simulink model "Model_3RC_P0"  (R2022b)
settings: Solver=FixedStepAuto  StartTime=0.0  StopTime=10000  FixedStep=1  RelTol=1e-3
undefined symbols (not defined in the file): epsilon, OCV, OCV_offset, R0, R1, R2, R3, SOC_levels, tau1, tau2, tau3
settings Model: Creator=frederikvanmaele  LastModifiedBy=AdministratorDevice
settings DebuggingCC: UnconnectedInputMsg=warning  UnconnectedOutputMsg=warning  UnconnectedLineMsg=warning
settings ModelReferenceCC: EnableRefExpFcnMdlSchedulingChecks=on
settings RTWCC: DLArmComputeVersion=19.05

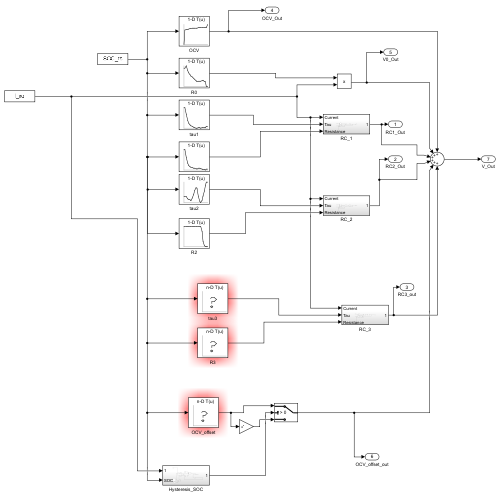
[thumbnail: Simulink's stored preview of the top-level diagram]
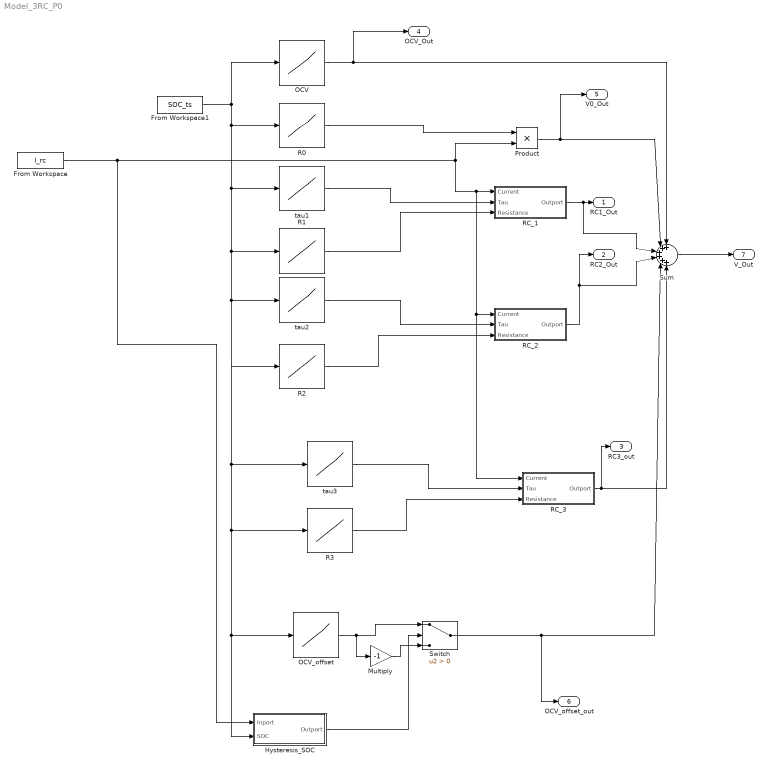
== system Model_3RC_P0 ==
  From Workspace : FromWorkspace  VariableName=I_rc
  From Workspace1 : FromWorkspace  VariableName=SOC_ts
  Hysteresis_SOC : Subsystem
  Multiply : Gain  Gain=-1
  OCV : Lookup_n-D  NumberOfTableDimensions=1  BreakpointsForDimension1=SOC_levels  BeginIndexSearchUsingPreviousIndexResult=on  Table=OCV  UseLastTableValue=on  InternalRulePriority=Speed  OutDataTypeStr=Inherit: Inherit via back propagation  RndMeth=Simplest
  OCV_offset : Lookup_n-D  NumberOfTableDimensions=1  BreakpointsForDimension1=SOC_levels  Table=OCV_offset  InternalRulePriority=Speed  RndMeth=Simplest
  Product : Product
  R0 : Lookup_n-D  NumberOfTableDimensions=1  BreakpointsForDimension1=SOC_levels  BeginIndexSearchUsingPreviousIndexResult=on  Table=R0  ExtrapMethod=Clip  UseLastTableValue=on  InternalRulePriority=Speed  RndMeth=Simplest
  R1 : Lookup_n-D  NumberOfTableDimensions=1  BreakpointsForDimension1=SOC_levels  BeginIndexSearchUsingPreviousIndexResult=on  Table=R1  ExtrapMethod=Clip  UseLastTableValue=on  InternalRulePriority=Speed  RndMeth=Simplest
  R2 : Lookup_n-D  NumberOfTableDimensions=1  BreakpointsForDimension1=SOC_levels  BeginIndexSearchUsingPreviousIndexResult=on  Table=R2  ExtrapMethod=Clip  UseLastTableValue=on  InternalRulePriority=Speed  RndMeth=Simplest
  R3 : Lookup_n-D  NumberOfTableDimensions=1  BreakpointsForDimension1=SOC_levels  BeginIndexSearchUsingPreviousIndexResult=on  Table=R3  ExtrapMethod=Clip  UseLastTableValue=on  InternalRulePriority=Speed  RndMeth=Simplest
  RC_1 : Subsystem
  RC_2 : Subsystem
  RC_3 : Subsystem
  Sum : Sum  Inputs=++++++
  Switch : Switch  Criteria=u2 > Threshold  SaturateOnIntegerOverflow=off  InputSameDT=off
  tau1 : Lookup_n-D  NumberOfTableDimensions=1  BreakpointsForDimension1=SOC_levels  BeginIndexSearchUsingPreviousIndexResult=on  Table=tau1  ExtrapMethod=Clip  UseLastTableValue=on  InternalRulePriority=Speed  RndMeth=Simplest
  tau2 : Lookup_n-D  NumberOfTableDimensions=1  BreakpointsForDimension1=SOC_levels  BeginIndexSearchUsingPreviousIndexResult=on  Table=tau2  ExtrapMethod=Clip  UseLastTableValue=on  InternalRulePriority=Speed  RndMeth=Simplest
  tau3 : Lookup_n-D  NumberOfTableDimensions=1  BreakpointsForDimension1=SOC_levels  BeginIndexSearchUsingPreviousIndexResult=on  Table=tau3  ExtrapMethod=Clip  UseLastTableValue=on  InternalRulePriority=Speed  RndMeth=Simplest
  RC1_Out : Outport
  RC2_Out : Outport  Port=2
  RC3_out : Outport  Port=3
  OCV_Out : Outport  Port=4
  V0_Out : Outport  Port=5
  OCV_offset_out : Outport  Port=6
  V_Out : Outport  Port=7
  wires:
  R1/1 -> RC_1/3(Resistance)
  tau1/1 -> RC_1/2(Tau)
  RC_1/1(Outport) -> Sum/3, RC1_Out/1
  R2/1 -> RC_2/3(Resistance)
  RC_2/1(Outport) -> RC2_Out/1, Sum/4
  OCV/1 -> OCV_Out/1, Sum/1
  Sum/1 -> V_Out/1
  From Workspace1/1 -> tau3/1, R3/1, Hysteresis_SOC/2(SOC), OCV_offset/1, R1/1, R2/1, tau2/1, tau1/1, R0/1, OCV/1
  R0/1 -> Product/1
  Product/1 -> V0_Out/1, Sum/2
  tau2/1 -> RC_2/2(Tau)
  Multiply/1 -> Switch/3
  Hysteresis_SOC/1(Outport) -> Switch/2
  OCV_offset/1 -> Multiply/1, Switch/1
  Switch/1 -> Sum/5, OCV_offset_out/1
  R3/1 -> RC_3/3(Resistance)
  tau3/1 -> RC_3/2(Tau)
  From Workspace/1 -> Hysteresis_SOC/1(Inport), RC_1/1(Current), RC_3/1(Current), RC_2/1(Current), Product/2
  RC_3/1(Outport) -> RC3_out/1, Sum/6

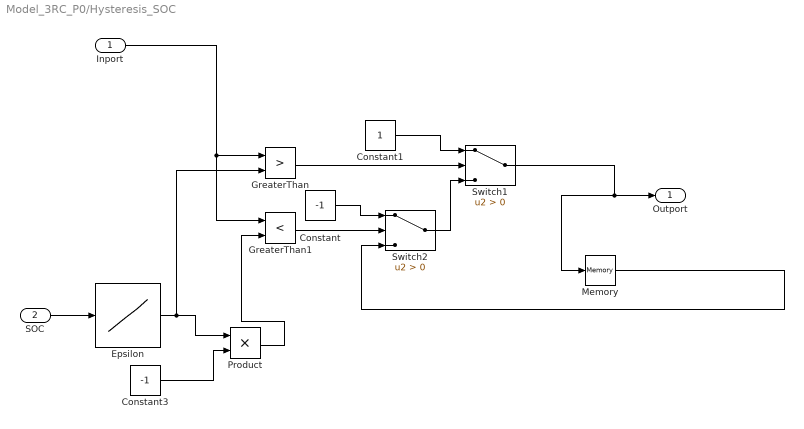
== system Model_3RC_P0/Hysteresis_SOC ==
  Inport : Inport
  SOC : Inport  Port=2
  Constant : Constant  Value=-1
  Constant1 : Constant
  Constant3 : Constant  Value=-1
  Epsilon : Lookup_n-D  NumberOfTableDimensions=1  BreakpointsForDimension1=SOC_levels  Table=epsilon  InternalRulePriority=Speed  RndMeth=Simplest
  GreaterThan : RelationalOperator  Operator=>  OutDataTypeStr=boolean  RndMeth=Simplest  InputSameDT=off
  GreaterThan1 : RelationalOperator  Operator=<  OutDataTypeStr=boolean  RndMeth=Simplest  InputSameDT=off
  Memory : Memory
  Product : Product
  Switch1 : Switch  Criteria=u2 > Threshold  SaturateOnIntegerOverflow=off  InputSameDT=off
  Switch2 : Switch  Criteria=u2 > Threshold  SaturateOnIntegerOverflow=off  InputSameDT=off
  Outport : Outport
  wires:
  GreaterThan1/1 -> Switch2/2
  Constant/1 -> Switch2/1
  Switch1/1 -> Outport/1, Memory/1
  Inport/1 -> GreaterThan1/1, GreaterThan/1
  Constant1/1 -> Switch1/1
  Switch2/1 -> Switch1/3
  GreaterThan/1 -> Switch1/2
  Memory/1 -> Switch2/3
  SOC/1 -> Epsilon/1
  Epsilon/1 -> GreaterThan/2, Product/1
  Constant3/1 -> Product/2
  Product/1 -> GreaterThan1/2

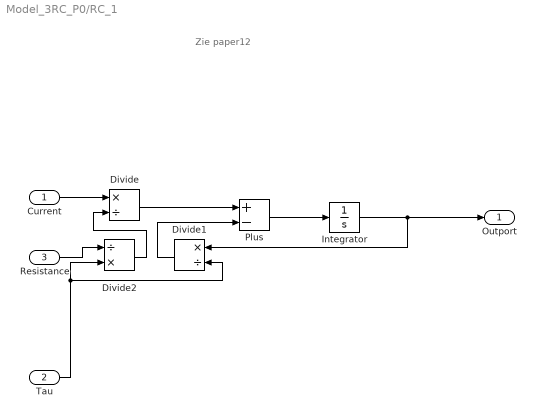
== system Model_3RC_P0/RC_1 ==
  note: Zie paper12
  Current : Inport
  Tau : Inport  Port=2
  Resistance : Inport  Port=3
  Divide : Product  Inputs=*/
  Divide1 : Product  Inputs=*/
  Divide2 : Product  Inputs=/*
  Integrator : Integrator
  Plus : Sum  Inputs=+-
  Outport : Outport
  wires:
  Tau/1 -> Divide2/2, Divide1/2
  Divide/1 -> Plus/1
  Plus/1 -> Integrator/1
  Current/1 -> Divide/1
  Divide1/1 -> Plus/2
  Resistance/1 -> Divide2/1
  Divide2/1 -> Divide/2
  Integrator/1 -> Divide1/1, Outport/1

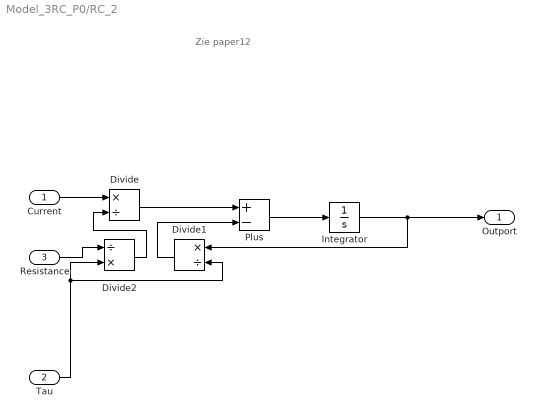
== system Model_3RC_P0/RC_2 ==
  note: Zie paper12
  Current : Inport
  Tau : Inport  Port=2
  Resistance : Inport  Port=3
  Divide : Product  Inputs=*/
  Divide1 : Product  Inputs=*/
  Divide2 : Product  Inputs=/*
  Integrator : Integrator
  Plus : Sum  Inputs=+-
  Outport : Outport
  wires:
  Tau/1 -> Divide2/2, Divide1/2
  Divide/1 -> Plus/1
  Plus/1 -> Integrator/1
  Current/1 -> Divide/1
  Divide1/1 -> Plus/2
  Resistance/1 -> Divide2/1
  Divide2/1 -> Divide/2
  Integrator/1 -> Divide1/1, Outport/1

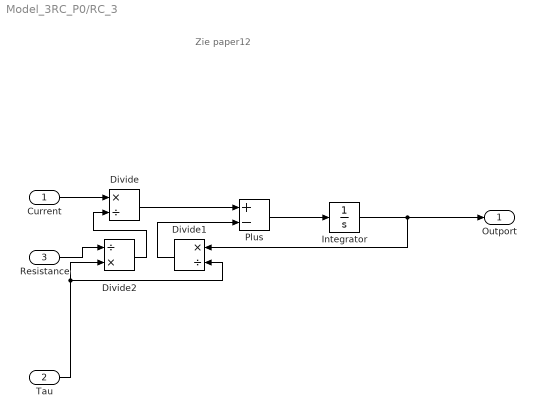
== system Model_3RC_P0/RC_3 ==
  note: Zie paper12
  Current : Inport
  Tau : Inport  Port=2
  Resistance : Inport  Port=3
  Divide : Product  Inputs=*/
  Divide1 : Product  Inputs=*/
  Divide2 : Product  Inputs=/*
  Integrator : Integrator
  Plus : Sum  Inputs=+-
  Outport : Outport
  wires:
  Tau/1 -> Divide2/2, Divide1/2
  Divide/1 -> Plus/1
  Plus/1 -> Integrator/1
  Current/1 -> Divide/1
  Divide1/1 -> Plus/2
  Resistance/1 -> Divide2/1
  Divide2/1 -> Divide/2
  Integrator/1 -> Divide1/1, Outport/1
